simulink model "ensembleSNN_simulink"  (R2019a)
settings: Solver=FixedStepAuto  StartTime=0.0  StopTime=12  FixedStep=0.001  RelTol=1e-3
libraries: simulink x2, dspsigops x1
(part 2 of 3)

== system ensembleSNN_simulink/izhiekvichNeuron10/u' switch ==
  In1 : Inport
  In2 : Inport  Port=2
  In3 : Inport  Port=3
  Switch Delay - 3 : Delay  DelayLength=3
  Switch4 : Switch  Criteria=u2 > Threshold  Threshold=30
  Out1 : Outport  VectorParamsAs1DForOutWhenUnconnected=on
  wires:
  In2/1 -> Switch4/2
  Switch4/1 -> Switch Delay - 3/1
  In1/1 -> Switch4/1
  Switch Delay - 3/1 -> Out1/1
  In3/1 -> Switch4/3

== system ensembleSNN_simulink/izhiekvichNeuron10/v + [0.04v2 +5v - u + j +140 ==
  In1 : Inport
  J : Inport  Port=2
  Add : Sum
  Add Delay - 2 : Delay
  Out1 : Outport  VectorParamsAs1DForOutWhenUnconnected=on
  wires:
  Add Delay - 2/1 -> Out1/1
  Add/1 -> Add Delay - 2/1
  In1/1 -> Add/1
  J/1 -> Add/2

== system ensembleSNN_simulink/izhiekvichNeuron10/v' switch ==
  In1 : Inport
  In2 : Inport  Port=2
  In3 : Inport  Port=3
  Switch Delay - 3 : Delay  DelayLength=3
  Switch4 : Switch  Criteria=u2 > Threshold  Threshold=30
  J : Outport  VectorParamsAs1DForOutWhenUnconnected=on
  wires:
  In2/1 -> Switch4/2
  Switch4/1 -> Switch Delay - 3/1
  In1/1 -> Switch4/1
  Switch Delay - 3/1 -> J/1
  In3/1 -> Switch4/3

== system ensembleSNN_simulink/izhiekvichNeuron10/v^2 ==
  J : Inport
  In2 : Inport  Port=2
  Mult Delay - 2 : Delay  DelayLength=1
  Product1 : Product
  Out1 : Outport  VectorParamsAs1DForOutWhenUnconnected=on
  wires:
  Product1/1 -> Mult Delay - 2/1
  In2/1 -> Product1/2
  J/1 -> Product1/1
  Mult Delay - 2/1 -> Out1/1

== system ensembleSNN_simulink/izhiekvichNeuron11/0.04v2 +5v - u ==
  In1 : Inport
  In2 : Inport  Port=2
  Subtract : Sum  Inputs=+-
  Subtract Delay - 1 : Delay  DelayLength=1
  Out1 : Outport  VectorParamsAs1DForOutWhenUnconnected=on
  wires:
  In1/1 -> Subtract/1
  Subtract/1 -> Subtract Delay - 1/1
  Subtract Delay - 1/1 -> Out1/1
  In2/1 -> Subtract/2

== system ensembleSNN_simulink/izhiekvichNeuron11/0.04v2 +5v - u + j +140 ==
  In1 : Inport
  J : Inport  Port=2
  Add : Sum
  Add Delay - 2 : Delay
  Out1 : Outport  VectorParamsAs1DForOutWhenUnconnected=on
  wires:
  Add Delay - 2/1 -> Out1/1
  Add/1 -> Add Delay - 2/1
  In1/1 -> Add/1
  J/1 -> Add/2

== system ensembleSNN_simulink/izhiekvichNeuron11/0.04v^2 ==
  In1 : Inport
  In2 : Inport  Port=2
  Mult Delay - 1 : Delay  DelayLength=1
  Product1 : Product
  Out1 : Outport  VectorParamsAs1DForOutWhenUnconnected=on
  wires:
  Product1/1 -> Mult Delay - 1/1
  Mult Delay - 1/1 -> Out1/1
  In2/1 -> Product1/2
  In1/1 -> Product1/1

== system ensembleSNN_simulink/izhiekvichNeuron11/0.04v^2 +5v ==
  In1 : Inport
  In2 : Inport  Port=2
  Add : Sum
  Add Delay - 2 : Delay
  Out1 : Outport  VectorParamsAs1DForOutWhenUnconnected=on
  wires:
  Add Delay - 2/1 -> Out1/1
  Add/1 -> Add Delay - 2/1
  In1/1 -> Add/1
  In2/1 -> Add/2

== system ensembleSNN_simulink/izhiekvichNeuron11/5v ==
  J : Inport
  In2 : Inport  Port=2
  Mult Delay - 1 : Delay  DelayLength=1
  Product1 : Product
  Out1 : Outport  VectorParamsAs1DForOutWhenUnconnected=on
  wires:
  Product1/1 -> Mult Delay - 1/1
  Mult Delay - 1/1 -> Out1/1
  In2/1 -> Product1/2
  J/1 -> Product1/1

== system ensembleSNN_simulink/izhiekvichNeuron11/a(bv-u) ==
  In1 : Inport
  In2 : Inport  Port=2
  Mult Delay - 1 : Delay  DelayLength=1
  Product1 : Product
  Out1 : Outport  VectorParamsAs1DForOutWhenUnconnected=on
  wires:
  Product1/1 -> Mult Delay - 1/1
  Mult Delay - 1/1 -> Out1/1
  In2/1 -> Product1/2
  In1/1 -> Product1/1

== system ensembleSNN_simulink/izhiekvichNeuron11/bv ==
  In1 : Inport
  J : Inport  Port=2
  Mult Delay - 1 : Delay  DelayLength=1
  Product1 : Product
  Out1 : Outport  VectorParamsAs1DForOutWhenUnconnected=on
  wires:
  Product1/1 -> Mult Delay - 1/1
  Mult Delay - 1/1 -> Out1/1
  J/1 -> Product1/2
  In1/1 -> Product1/1

== system ensembleSNN_simulink/izhiekvichNeuron11/bv - u ==
  In1 : Inport
  In2 : Inport  Port=2
  Subtract : Sum  Inputs=+-
  Subtract Delay - 1 : Delay  DelayLength=1
  Out1 : Outport  VectorParamsAs1DForOutWhenUnconnected=on
  wires:
  In1/1 -> Subtract/1
  Subtract/1 -> Subtract Delay - 1/1
  Subtract Delay - 1/1 -> Out1/1
  In2/1 -> Subtract/2

== system ensembleSNN_simulink/izhiekvichNeuron11/j + 140 ==
  In1 : Inport
  J : Inport  Port=2
  Add : Sum
  Add Delay - 2 : Delay
  Out1 : Outport  VectorParamsAs1DForOutWhenUnconnected=on
  wires:
  Add Delay - 2/1 -> Out1/1
  Add/1 -> Add Delay - 2/1
  In1/1 -> Add/1
  J/1 -> Add/2

== system ensembleSNN_simulink/izhiekvichNeuron11/u + a(bv-u) ==
  In1 : Inport
  In2 : Inport  Port=2
  Add : Sum
  Add Delay - 2 : Delay
  Out1 : Outport  VectorParamsAs1DForOutWhenUnconnected=on
  wires:
  Add Delay - 2/1 -> Out1/1
  Add/1 -> Add Delay - 2/1
  In1/1 -> Add/1
  In2/1 -> Add/2

== system ensembleSNN_simulink/izhiekvichNeuron11/u' + d ==
  In1 : Inport
  In2 : Inport  Port=2
  Add : Sum
  Add Delay - 2 : Delay
  Out1 : Outport  VectorParamsAs1DForOutWhenUnconnected=on
  wires:
  Add Delay - 2/1 -> Out1/1
  Add/1 -> Add Delay - 2/1
  In1/1 -> Add/1
  In2/1 -> Add/2

== system ensembleSNN_simulink/izhiekvichNeuron11/u' switch ==
  In1 : Inport
  In2 : Inport  Port=2
  In3 : Inport  Port=3
  Switch Delay - 3 : Delay  DelayLength=3
  Switch4 : Switch  Criteria=u2 > Threshold  Threshold=30
  Out1 : Outport  VectorParamsAs1DForOutWhenUnconnected=on
  wires:
  In2/1 -> Switch4/2
  Switch4/1 -> Switch Delay - 3/1
  In1/1 -> Switch4/1
  Switch Delay - 3/1 -> Out1/1
  In3/1 -> Switch4/3

== system ensembleSNN_simulink/izhiekvichNeuron11/v + [0.04v2 +5v - u + j +140 ==
  In1 : Inport
  J : Inport  Port=2
  Add : Sum
  Add Delay - 2 : Delay
  Out1 : Outport  VectorParamsAs1DForOutWhenUnconnected=on
  wires:
  Add Delay - 2/1 -> Out1/1
  Add/1 -> Add Delay - 2/1
  In1/1 -> Add/1
  J/1 -> Add/2

== system ensembleSNN_simulink/izhiekvichNeuron11/v' switch ==
  In1 : Inport
  In2 : Inport  Port=2
  In3 : Inport  Port=3
  Switch Delay - 3 : Delay  DelayLength=3
  Switch4 : Switch  Criteria=u2 > Threshold  Threshold=30
  J : Outport  VectorParamsAs1DForOutWhenUnconnected=on
  wires:
  In2/1 -> Switch4/2
  Switch4/1 -> Switch Delay - 3/1
  In1/1 -> Switch4/1
  Switch Delay - 3/1 -> J/1
  In3/1 -> Switch4/3

== system ensembleSNN_simulink/izhiekvichNeuron11/v^2 ==
  J : Inport
  In2 : Inport  Port=2
  Mult Delay - 2 : Delay  DelayLength=1
  Product1 : Product
  Out1 : Outport  VectorParamsAs1DForOutWhenUnconnected=on
  wires:
  Product1/1 -> Mult Delay - 2/1
  In2/1 -> Product1/2
  J/1 -> Product1/1
  Mult Delay - 2/1 -> Out1/1

== system ensembleSNN_simulink/izhiekvichNeuron12/0.04v2 +5v - u ==
  In1 : Inport
  In2 : Inport  Port=2
  Subtract : Sum  Inputs=+-
  Subtract Delay - 1 : Delay  DelayLength=1
  Out1 : Outport  VectorParamsAs1DForOutWhenUnconnected=on
  wires:
  In1/1 -> Subtract/1
  Subtract/1 -> Subtract Delay - 1/1
  Subtract Delay - 1/1 -> Out1/1
  In2/1 -> Subtract/2

== system ensembleSNN_simulink/izhiekvichNeuron12/0.04v2 +5v - u + j +140 ==
  In1 : Inport
  J : Inport  Port=2
  Add : Sum
  Add Delay - 2 : Delay
  Out1 : Outport  VectorParamsAs1DForOutWhenUnconnected=on
  wires:
  Add Delay - 2/1 -> Out1/1
  Add/1 -> Add Delay - 2/1
  In1/1 -> Add/1
  J/1 -> Add/2

== system ensembleSNN_simulink/izhiekvichNeuron12/0.04v^2 ==
  In1 : Inport
  In2 : Inport  Port=2
  Mult Delay - 1 : Delay  DelayLength=1
  Product1 : Product
  Out1 : Outport  VectorParamsAs1DForOutWhenUnconnected=on
  wires:
  Product1/1 -> Mult Delay - 1/1
  Mult Delay - 1/1 -> Out1/1
  In2/1 -> Product1/2
  In1/1 -> Product1/1

== system ensembleSNN_simulink/izhiekvichNeuron12/0.04v^2 +5v ==
  In1 : Inport
  In2 : Inport  Port=2
  Add : Sum
  Add Delay - 2 : Delay
  Out1 : Outport  VectorParamsAs1DForOutWhenUnconnected=on
  wires:
  Add Delay - 2/1 -> Out1/1
  Add/1 -> Add Delay - 2/1
  In1/1 -> Add/1
  In2/1 -> Add/2

== system ensembleSNN_simulink/izhiekvichNeuron12/5v ==
  J : Inport
  In2 : Inport  Port=2
  Mult Delay - 1 : Delay  DelayLength=1
  Product1 : Product
  Out1 : Outport  VectorParamsAs1DForOutWhenUnconnected=on
  wires:
  Product1/1 -> Mult Delay - 1/1
  Mult Delay - 1/1 -> Out1/1
  In2/1 -> Product1/2
  J/1 -> Product1/1

== system ensembleSNN_simulink/izhiekvichNeuron12/a(bv-u) ==
  In1 : Inport
  In2 : Inport  Port=2
  Mult Delay - 1 : Delay  DelayLength=1
  Product1 : Product
  Out1 : Outport  VectorParamsAs1DForOutWhenUnconnected=on
  wires:
  Product1/1 -> Mult Delay - 1/1
  Mult Delay - 1/1 -> Out1/1
  In2/1 -> Product1/2
  In1/1 -> Product1/1

== system ensembleSNN_simulink/izhiekvichNeuron12/bv ==
  In1 : Inport
  J : Inport  Port=2
  Mult Delay - 1 : Delay  DelayLength=1
  Product1 : Product
  Out1 : Outport  VectorParamsAs1DForOutWhenUnconnected=on
  wires:
  Product1/1 -> Mult Delay - 1/1
  Mult Delay - 1/1 -> Out1/1
  J/1 -> Product1/2
  In1/1 -> Product1/1

== system ensembleSNN_simulink/izhiekvichNeuron12/bv - u ==
  In1 : Inport
  In2 : Inport  Port=2
  Subtract : Sum  Inputs=+-
  Subtract Delay - 1 : Delay  DelayLength=1
  Out1 : Outport  VectorParamsAs1DForOutWhenUnconnected=on
  wires:
  In1/1 -> Subtract/1
  Subtract/1 -> Subtract Delay - 1/1
  Subtract Delay - 1/1 -> Out1/1
  In2/1 -> Subtract/2

== system ensembleSNN_simulink/izhiekvichNeuron12/j + 140 ==
  In1 : Inport
  J : Inport  Port=2
  Add : Sum
  Add Delay - 2 : Delay
  Out1 : Outport  VectorParamsAs1DForOutWhenUnconnected=on
  wires:
  Add Delay - 2/1 -> Out1/1
  Add/1 -> Add Delay - 2/1
  In1/1 -> Add/1
  J/1 -> Add/2

== system ensembleSNN_simulink/izhiekvichNeuron12/u + a(bv-u) ==
  In1 : Inport
  In2 : Inport  Port=2
  Add : Sum
  Add Delay - 2 : Delay
  Out1 : Outport  VectorParamsAs1DForOutWhenUnconnected=on
  wires:
  Add Delay - 2/1 -> Out1/1
  Add/1 -> Add Delay - 2/1
  In1/1 -> Add/1
  In2/1 -> Add/2

== system ensembleSNN_simulink/izhiekvichNeuron12/u' + d ==
  In1 : Inport
  In2 : Inport  Port=2
  Add : Sum
  Add Delay - 2 : Delay
  Out1 : Outport  VectorParamsAs1DForOutWhenUnconnected=on
  wires:
  Add Delay - 2/1 -> Out1/1
  Add/1 -> Add Delay - 2/1
  In1/1 -> Add/1
  In2/1 -> Add/2

== system ensembleSNN_simulink/izhiekvichNeuron12/u' switch ==
  In1 : Inport
  In2 : Inport  Port=2
  In3 : Inport  Port=3
  Switch Delay - 3 : Delay  DelayLength=3
  Switch4 : Switch  Criteria=u2 > Threshold  Threshold=30
  Out1 : Outport  VectorParamsAs1DForOutWhenUnconnected=on
  wires:
  In2/1 -> Switch4/2
  Switch4/1 -> Switch Delay - 3/1
  In1/1 -> Switch4/1
  Switch Delay - 3/1 -> Out1/1
  In3/1 -> Switch4/3

== system ensembleSNN_simulink/izhiekvichNeuron12/v + [0.04v2 +5v - u + j +140 ==
  In1 : Inport
  J : Inport  Port=2
  Add : Sum
  Add Delay - 2 : Delay
  Out1 : Outport  VectorParamsAs1DForOutWhenUnconnected=on
  wires:
  Add Delay - 2/1 -> Out1/1
  Add/1 -> Add Delay - 2/1
  In1/1 -> Add/1
  J/1 -> Add/2

== system ensembleSNN_simulink/izhiekvichNeuron12/v' switch ==
  In1 : Inport
  In2 : Inport  Port=2
  In3 : Inport  Port=3
  Switch Delay - 3 : Delay  DelayLength=3
  Switch4 : Switch  Criteria=u2 > Threshold  Threshold=30
  J : Outport  VectorParamsAs1DForOutWhenUnconnected=on
  wires:
  In2/1 -> Switch4/2
  Switch4/1 -> Switch Delay - 3/1
  In1/1 -> Switch4/1
  Switch Delay - 3/1 -> J/1
  In3/1 -> Switch4/3

== system ensembleSNN_simulink/izhiekvichNeuron12/v^2 ==
  J : Inport
  In2 : Inport  Port=2
  Mult Delay - 2 : Delay  DelayLength=1
  Product1 : Product
  Out1 : Outport  VectorParamsAs1DForOutWhenUnconnected=on
  wires:
  Product1/1 -> Mult Delay - 2/1
  In2/1 -> Product1/2
  J/1 -> Product1/1
  Mult Delay - 2/1 -> Out1/1

== system ensembleSNN_simulink/izhiekvichNeuron13/0.04v2 +5v - u ==
  In1 : Inport
  In2 : Inport  Port=2
  Subtract : Sum  Inputs=+-
  Subtract Delay - 1 : Delay  DelayLength=1
  Out1 : Outport  VectorParamsAs1DForOutWhenUnconnected=on
  wires:
  In1/1 -> Subtract/1
  Subtract/1 -> Subtract Delay - 1/1
  Subtract Delay - 1/1 -> Out1/1
  In2/1 -> Subtract/2

== system ensembleSNN_simulink/izhiekvichNeuron13/0.04v2 +5v - u + j +140 ==
  In1 : Inport
  J : Inport  Port=2
  Add : Sum
  Add Delay - 2 : Delay
  Out1 : Outport  VectorParamsAs1DForOutWhenUnconnected=on
  wires:
  Add Delay - 2/1 -> Out1/1
  Add/1 -> Add Delay - 2/1
  In1/1 -> Add/1
  J/1 -> Add/2

== system ensembleSNN_simulink/izhiekvichNeuron13/0.04v^2 ==
  In1 : Inport
  In2 : Inport  Port=2
  Mult Delay - 1 : Delay  DelayLength=1
  Product1 : Product
  Out1 : Outport  VectorParamsAs1DForOutWhenUnconnected=on
  wires:
  Product1/1 -> Mult Delay - 1/1
  Mult Delay - 1/1 -> Out1/1
  In2/1 -> Product1/2
  In1/1 -> Product1/1

== system ensembleSNN_simulink/izhiekvichNeuron13/0.04v^2 +5v ==
  In1 : Inport
  In2 : Inport  Port=2
  Add : Sum
  Add Delay - 2 : Delay
  Out1 : Outport  VectorParamsAs1DForOutWhenUnconnected=on
  wires:
  Add Delay - 2/1 -> Out1/1
  Add/1 -> Add Delay - 2/1
  In1/1 -> Add/1
  In2/1 -> Add/2

== system ensembleSNN_simulink/izhiekvichNeuron13/5v ==
  J : Inport
  In2 : Inport  Port=2
  Mult Delay - 1 : Delay  DelayLength=1
  Product1 : Product
  Out1 : Outport  VectorParamsAs1DForOutWhenUnconnected=on
  wires:
  Product1/1 -> Mult Delay - 1/1
  Mult Delay - 1/1 -> Out1/1
  In2/1 -> Product1/2
  J/1 -> Product1/1

== system ensembleSNN_simulink/izhiekvichNeuron13/a(bv-u) ==
  In1 : Inport
  In2 : Inport  Port=2
  Mult Delay - 1 : Delay  DelayLength=1
  Product1 : Product
  Out1 : Outport  VectorParamsAs1DForOutWhenUnconnected=on
  wires:
  Product1/1 -> Mult Delay - 1/1
  Mult Delay - 1/1 -> Out1/1
  In2/1 -> Product1/2
  In1/1 -> Product1/1

== system ensembleSNN_simulink/izhiekvichNeuron13/bv ==
  In1 : Inport
  J : Inport  Port=2
  Mult Delay - 1 : Delay  DelayLength=1
  Product1 : Product
  Out1 : Outport  VectorParamsAs1DForOutWhenUnconnected=on
  wires:
  Product1/1 -> Mult Delay - 1/1
  Mult Delay - 1/1 -> Out1/1
  J/1 -> Product1/2
  In1/1 -> Product1/1

== system ensembleSNN_simulink/izhiekvichNeuron13/bv - u ==
  In1 : Inport
  In2 : Inport  Port=2
  Subtract : Sum  Inputs=+-
  Subtract Delay - 1 : Delay  DelayLength=1
  Out1 : Outport  VectorParamsAs1DForOutWhenUnconnected=on
  wires:
  In1/1 -> Subtract/1
  Subtract/1 -> Subtract Delay - 1/1
  Subtract Delay - 1/1 -> Out1/1
  In2/1 -> Subtract/2

== system ensembleSNN_simulink/izhiekvichNeuron13/j + 140 ==
  In1 : Inport
  J : Inport  Port=2
  Add : Sum
  Add Delay - 2 : Delay
  Out1 : Outport  VectorParamsAs1DForOutWhenUnconnected=on
  wires:
  Add Delay - 2/1 -> Out1/1
  Add/1 -> Add Delay - 2/1
  In1/1 -> Add/1
  J/1 -> Add/2

== system ensembleSNN_simulink/izhiekvichNeuron13/u + a(bv-u) ==
  In1 : Inport
  In2 : Inport  Port=2
  Add : Sum
  Add Delay - 2 : Delay
  Out1 : Outport  VectorParamsAs1DForOutWhenUnconnected=on
  wires:
  Add Delay - 2/1 -> Out1/1
  Add/1 -> Add Delay - 2/1
  In1/1 -> Add/1
  In2/1 -> Add/2

== system ensembleSNN_simulink/izhiekvichNeuron13/u' + d ==
  In1 : Inport
  In2 : Inport  Port=2
  Add : Sum
  Add Delay - 2 : Delay
  Out1 : Outport  VectorParamsAs1DForOutWhenUnconnected=on
  wires:
  Add Delay - 2/1 -> Out1/1
  Add/1 -> Add Delay - 2/1
  In1/1 -> Add/1
  In2/1 -> Add/2

== system ensembleSNN_simulink/izhiekvichNeuron13/u' switch ==
  In1 : Inport
  In2 : Inport  Port=2
  In3 : Inport  Port=3
  Switch Delay - 3 : Delay  DelayLength=3
  Switch4 : Switch  Criteria=u2 > Threshold  Threshold=30
  Out1 : Outport  VectorParamsAs1DForOutWhenUnconnected=on
  wires:
  In2/1 -> Switch4/2
  Switch4/1 -> Switch Delay - 3/1
  In1/1 -> Switch4/1
  Switch Delay - 3/1 -> Out1/1
  In3/1 -> Switch4/3

== system ensembleSNN_simulink/izhiekvichNeuron13/v + [0.04v2 +5v - u + j +140 ==
  In1 : Inport
  J : Inport  Port=2
  Add : Sum
  Add Delay - 2 : Delay
  Out1 : Outport  VectorParamsAs1DForOutWhenUnconnected=on
  wires:
  Add Delay - 2/1 -> Out1/1
  Add/1 -> Add Delay - 2/1
  In1/1 -> Add/1
  J/1 -> Add/2

== system ensembleSNN_simulink/izhiekvichNeuron13/v' switch ==
  In1 : Inport
  In2 : Inport  Port=2
  In3 : Inport  Port=3
  Switch Delay - 3 : Delay  DelayLength=3
  Switch4 : Switch  Criteria=u2 > Threshold  Threshold=30
  J : Outport  VectorParamsAs1DForOutWhenUnconnected=on
  wires:
  In2/1 -> Switch4/2
  Switch4/1 -> Switch Delay - 3/1
  In1/1 -> Switch4/1
  Switch Delay - 3/1 -> J/1
  In3/1 -> Switch4/3

== system ensembleSNN_simulink/izhiekvichNeuron13/v^2 ==
  J : Inport
  In2 : Inport  Port=2
  Mult Delay - 2 : Delay  DelayLength=1
  Product1 : Product
  Out1 : Outport  VectorParamsAs1DForOutWhenUnconnected=on
  wires:
  Product1/1 -> Mult Delay - 2/1
  In2/1 -> Product1/2
  J/1 -> Product1/1
  Mult Delay - 2/1 -> Out1/1

== system ensembleSNN_simulink/izhiekvichNeuron14/0.04v2 +5v - u ==
  In1 : Inport
  In2 : Inport  Port=2
  Subtract : Sum  Inputs=+-
  Subtract Delay - 1 : Delay  DelayLength=1
  Out1 : Outport  VectorParamsAs1DForOutWhenUnconnected=on
  wires:
  In1/1 -> Subtract/1
  Subtract/1 -> Subtract Delay - 1/1
  Subtract Delay - 1/1 -> Out1/1
  In2/1 -> Subtract/2

== system ensembleSNN_simulink/izhiekvichNeuron14/0.04v2 +5v - u + j +140 ==
  In1 : Inport
  J : Inport  Port=2
  Add : Sum
  Add Delay - 2 : Delay
  Out1 : Outport  VectorParamsAs1DForOutWhenUnconnected=on
  wires:
  Add Delay - 2/1 -> Out1/1
  Add/1 -> Add Delay - 2/1
  In1/1 -> Add/1
  J/1 -> Add/2

== system ensembleSNN_simulink/izhiekvichNeuron14/0.04v^2 ==
  In1 : Inport
  In2 : Inport  Port=2
  Mult Delay - 1 : Delay  DelayLength=1
  Product1 : Product
  Out1 : Outport  VectorParamsAs1DForOutWhenUnconnected=on
  wires:
  Product1/1 -> Mult Delay - 1/1
  Mult Delay - 1/1 -> Out1/1
  In2/1 -> Product1/2
  In1/1 -> Product1/1

== system ensembleSNN_simulink/izhiekvichNeuron14/0.04v^2 +5v ==
  In1 : Inport
  In2 : Inport  Port=2
  Add : Sum
  Add Delay - 2 : Delay
  Out1 : Outport  VectorParamsAs1DForOutWhenUnconnected=on
  wires:
  Add Delay - 2/1 -> Out1/1
  Add/1 -> Add Delay - 2/1
  In1/1 -> Add/1
  In2/1 -> Add/2

== system ensembleSNN_simulink/izhiekvichNeuron14/5v ==
  J : Inport
  In2 : Inport  Port=2
  Mult Delay - 1 : Delay  DelayLength=1
  Product1 : Product
  Out1 : Outport  VectorParamsAs1DForOutWhenUnconnected=on
  wires:
  Product1/1 -> Mult Delay - 1/1
  Mult Delay - 1/1 -> Out1/1
  In2/1 -> Product1/2
  J/1 -> Product1/1

== system ensembleSNN_simulink/izhiekvichNeuron14/a(bv-u) ==
  In1 : Inport
  In2 : Inport  Port=2
  Mult Delay - 1 : Delay  DelayLength=1
  Product1 : Product
  Out1 : Outport  VectorParamsAs1DForOutWhenUnconnected=on
  wires:
  Product1/1 -> Mult Delay - 1/1
  Mult Delay - 1/1 -> Out1/1
  In2/1 -> Product1/2
  In1/1 -> Product1/1

== system ensembleSNN_simulink/izhiekvichNeuron14/bv ==
  In1 : Inport
  J : Inport  Port=2
  Mult Delay - 1 : Delay  DelayLength=1
  Product1 : Product
  Out1 : Outport  VectorParamsAs1DForOutWhenUnconnected=on
  wires:
  Product1/1 -> Mult Delay - 1/1
  Mult Delay - 1/1 -> Out1/1
  J/1 -> Product1/2
  In1/1 -> Product1/1

== system ensembleSNN_simulink/izhiekvichNeuron14/bv - u ==
  In1 : Inport
  In2 : Inport  Port=2
  Subtract : Sum  Inputs=+-
  Subtract Delay - 1 : Delay  DelayLength=1
  Out1 : Outport  VectorParamsAs1DForOutWhenUnconnected=on
  wires:
  In1/1 -> Subtract/1
  Subtract/1 -> Subtract Delay - 1/1
  Subtract Delay - 1/1 -> Out1/1
  In2/1 -> Subtract/2

== system ensembleSNN_simulink/izhiekvichNeuron14/j + 140 ==
  In1 : Inport
  J : Inport  Port=2
  Add : Sum
  Add Delay - 2 : Delay
  Out1 : Outport  VectorParamsAs1DForOutWhenUnconnected=on
  wires:
  Add Delay - 2/1 -> Out1/1
  Add/1 -> Add Delay - 2/1
  In1/1 -> Add/1
  J/1 -> Add/2

== system ensembleSNN_simulink/izhiekvichNeuron14/u + a(bv-u) ==
  In1 : Inport
  In2 : Inport  Port=2
  Add : Sum
  Add Delay - 2 : Delay
  Out1 : Outport  VectorParamsAs1DForOutWhenUnconnected=on
  wires:
  Add Delay - 2/1 -> Out1/1
  Add/1 -> Add Delay - 2/1
  In1/1 -> Add/1
  In2/1 -> Add/2

== system ensembleSNN_simulink/izhiekvichNeuron14/u' + d ==
  In1 : Inport
  In2 : Inport  Port=2
  Add : Sum
  Add Delay - 2 : Delay
  Out1 : Outport  VectorParamsAs1DForOutWhenUnconnected=on
  wires:
  Add Delay - 2/1 -> Out1/1
  Add/1 -> Add Delay - 2/1
  In1/1 -> Add/1
  In2/1 -> Add/2

== system ensembleSNN_simulink/izhiekvichNeuron14/u' switch ==
  In1 : Inport
  In2 : Inport  Port=2
  In3 : Inport  Port=3
  Switch Delay - 3 : Delay  DelayLength=3
  Switch4 : Switch  Criteria=u2 > Threshold  Threshold=30
  Out1 : Outport  VectorParamsAs1DForOutWhenUnconnected=on
  wires:
  In2/1 -> Switch4/2
  Switch4/1 -> Switch Delay - 3/1
  In1/1 -> Switch4/1
  Switch Delay - 3/1 -> Out1/1
  In3/1 -> Switch4/3

== system ensembleSNN_simulink/izhiekvichNeuron14/v + [0.04v2 +5v - u + j +140 ==
  In1 : Inport
  J : Inport  Port=2
  Add : Sum
  Add Delay - 2 : Delay
  Out1 : Outport  VectorParamsAs1DForOutWhenUnconnected=on
  wires:
  Add Delay - 2/1 -> Out1/1
  Add/1 -> Add Delay - 2/1
  In1/1 -> Add/1
  J/1 -> Add/2

== system ensembleSNN_simulink/izhiekvichNeuron14/v' switch ==
  In1 : Inport
  In2 : Inport  Port=2
  In3 : Inport  Port=3
  Switch Delay - 3 : Delay  DelayLength=3
  Switch4 : Switch  Criteria=u2 > Threshold  Threshold=30
  J : Outport  VectorParamsAs1DForOutWhenUnconnected=on
  wires:
  In2/1 -> Switch4/2
  Switch4/1 -> Switch Delay - 3/1
  In1/1 -> Switch4/1
  Switch Delay - 3/1 -> J/1
  In3/1 -> Switch4/3

== system ensembleSNN_simulink/izhiekvichNeuron14/v^2 ==
  J : Inport
  In2 : Inport  Port=2
  Mult Delay - 2 : Delay  DelayLength=1
  Product1 : Product
  Out1 : Outport  VectorParamsAs1DForOutWhenUnconnected=on
  wires:
  Product1/1 -> Mult Delay - 2/1
  In2/1 -> Product1/2
  J/1 -> Product1/1
  Mult Delay - 2/1 -> Out1/1

== system ensembleSNN_simulink/izhiekvichNeuron15/0.04v2 +5v - u ==
  In1 : Inport
  In2 : Inport  Port=2
  Subtract : Sum  Inputs=+-
  Subtract Delay - 1 : Delay  DelayLength=1
  Out1 : Outport  VectorParamsAs1DForOutWhenUnconnected=on
  wires:
  In1/1 -> Subtract/1
  Subtract/1 -> Subtract Delay - 1/1
  Subtract Delay - 1/1 -> Out1/1
  In2/1 -> Subtract/2

== system ensembleSNN_simulink/izhiekvichNeuron15/0.04v2 +5v - u + j +140 ==
  In1 : Inport
  J : Inport  Port=2
  Add : Sum
  Add Delay - 2 : Delay
  Out1 : Outport  VectorParamsAs1DForOutWhenUnconnected=on
  wires:
  Add Delay - 2/1 -> Out1/1
  Add/1 -> Add Delay - 2/1
  In1/1 -> Add/1
  J/1 -> Add/2

== system ensembleSNN_simulink/izhiekvichNeuron15/0.04v^2 ==
  In1 : Inport
  In2 : Inport  Port=2
  Mult Delay - 1 : Delay  DelayLength=1
  Product1 : Product
  Out1 : Outport  VectorParamsAs1DForOutWhenUnconnected=on
  wires:
  Product1/1 -> Mult Delay - 1/1
  Mult Delay - 1/1 -> Out1/1
  In2/1 -> Product1/2
  In1/1 -> Product1/1

== system ensembleSNN_simulink/izhiekvichNeuron15/0.04v^2 +5v ==
  In1 : Inport
  In2 : Inport  Port=2
  Add : Sum
  Add Delay - 2 : Delay
  Out1 : Outport  VectorParamsAs1DForOutWhenUnconnected=on
  wires:
  Add Delay - 2/1 -> Out1/1
  Add/1 -> Add Delay - 2/1
  In1/1 -> Add/1
  In2/1 -> Add/2

== system ensembleSNN_simulink/izhiekvichNeuron15/5v ==
  J : Inport
  In2 : Inport  Port=2
  Mult Delay - 1 : Delay  DelayLength=1
  Product1 : Product
  Out1 : Outport  VectorParamsAs1DForOutWhenUnconnected=on
  wires:
  Product1/1 -> Mult Delay - 1/1
  Mult Delay - 1/1 -> Out1/1
  In2/1 -> Product1/2
  J/1 -> Product1/1

== system ensembleSNN_simulink/izhiekvichNeuron15/a(bv-u) ==
  In1 : Inport
  In2 : Inport  Port=2
  Mult Delay - 1 : Delay  DelayLength=1
  Product1 : Product
  Out1 : Outport  VectorParamsAs1DForOutWhenUnconnected=on
  wires:
  Product1/1 -> Mult Delay - 1/1
  Mult Delay - 1/1 -> Out1/1
  In2/1 -> Product1/2
  In1/1 -> Product1/1

== system ensembleSNN_simulink/izhiekvichNeuron15/bv ==
  In1 : Inport
  J : Inport  Port=2
  Mult Delay - 1 : Delay  DelayLength=1
  Product1 : Product
  Out1 : Outport  VectorParamsAs1DForOutWhenUnconnected=on
  wires:
  Product1/1 -> Mult Delay - 1/1
  Mult Delay - 1/1 -> Out1/1
  J/1 -> Product1/2
  In1/1 -> Product1/1

== system ensembleSNN_simulink/izhiekvichNeuron15/bv - u ==
  In1 : Inport
  In2 : Inport  Port=2
  Subtract : Sum  Inputs=+-
  Subtract Delay - 1 : Delay  DelayLength=1
  Out1 : Outport  VectorParamsAs1DForOutWhenUnconnected=on
  wires:
  In1/1 -> Subtract/1
  Subtract/1 -> Subtract Delay - 1/1
  Subtract Delay - 1/1 -> Out1/1
  In2/1 -> Subtract/2

== system ensembleSNN_simulink/izhiekvichNeuron15/j + 140 ==
  In1 : Inport
  J : Inport  Port=2
  Add : Sum
  Add Delay - 2 : Delay
  Out1 : Outport  VectorParamsAs1DForOutWhenUnconnected=on
  wires:
  Add Delay - 2/1 -> Out1/1
  Add/1 -> Add Delay - 2/1
  In1/1 -> Add/1
  J/1 -> Add/2

== system ensembleSNN_simulink/izhiekvichNeuron15/u + a(bv-u) ==
  In1 : Inport
  In2 : Inport  Port=2
  Add : Sum
  Add Delay - 2 : Delay
  Out1 : Outport  VectorParamsAs1DForOutWhenUnconnected=on
  wires:
  Add Delay - 2/1 -> Out1/1
  Add/1 -> Add Delay - 2/1
  In1/1 -> Add/1
  In2/1 -> Add/2

== system ensembleSNN_simulink/izhiekvichNeuron15/u' + d ==
  In1 : Inport
  In2 : Inport  Port=2
  Add : Sum
  Add Delay - 2 : Delay
  Out1 : Outport  VectorParamsAs1DForOutWhenUnconnected=on
  wires:
  Add Delay - 2/1 -> Out1/1
  Add/1 -> Add Delay - 2/1
  In1/1 -> Add/1
  In2/1 -> Add/2

== system ensembleSNN_simulink/izhiekvichNeuron15/u' switch ==
  In1 : Inport
  In2 : Inport  Port=2
  In3 : Inport  Port=3
  Switch Delay - 3 : Delay  DelayLength=3
  Switch4 : Switch  Criteria=u2 > Threshold  Threshold=30
  Out1 : Outport  VectorParamsAs1DForOutWhenUnconnected=on
  wires:
  In2/1 -> Switch4/2
  Switch4/1 -> Switch Delay - 3/1
  In1/1 -> Switch4/1
  Switch Delay - 3/1 -> Out1/1
  In3/1 -> Switch4/3

== system ensembleSNN_simulink/izhiekvichNeuron15/v + [0.04v2 +5v - u + j +140 ==
  In1 : Inport
  J : Inport  Port=2
  Add : Sum
  Add Delay - 2 : Delay
  Out1 : Outport  VectorParamsAs1DForOutWhenUnconnected=on
  wires:
  Add Delay - 2/1 -> Out1/1
  Add/1 -> Add Delay - 2/1
  In1/1 -> Add/1
  J/1 -> Add/2

== system ensembleSNN_simulink/izhiekvichNeuron15/v' switch ==
  In1 : Inport
  In2 : Inport  Port=2
  In3 : Inport  Port=3
  Switch Delay - 3 : Delay  DelayLength=3
  Switch4 : Switch  Criteria=u2 > Threshold  Threshold=30
  J : Outport  VectorParamsAs1DForOutWhenUnconnected=on
  wires:
  In2/1 -> Switch4/2
  Switch4/1 -> Switch Delay - 3/1
  In1/1 -> Switch4/1
  Switch Delay - 3/1 -> J/1
  In3/1 -> Switch4/3

== system ensembleSNN_simulink/izhiekvichNeuron15/v^2 ==
  J : Inport
  In2 : Inport  Port=2
  Mult Delay - 2 : Delay  DelayLength=1
  Product1 : Product
  Out1 : Outport  VectorParamsAs1DForOutWhenUnconnected=on
  wires:
  Product1/1 -> Mult Delay - 2/1
  In2/1 -> Product1/2
  J/1 -> Product1/1
  Mult Delay - 2/1 -> Out1/1

== system ensembleSNN_simulink/izhiekvichNeuron2/0.04v2 +5v - u ==
  In1 : Inport
  In2 : Inport  Port=2
  Subtract : Sum  Inputs=+-
  Subtract Delay - 1 : Delay  DelayLength=1
  Out1 : Outport  VectorParamsAs1DForOutWhenUnconnected=on
  wires:
  In1/1 -> Subtract/1
  Subtract/1 -> Subtract Delay - 1/1
  Subtract Delay - 1/1 -> Out1/1
  In2/1 -> Subtract/2

== system ensembleSNN_simulink/izhiekvichNeuron2/0.04v2 +5v - u + j +140 ==
  In1 : Inport
  J : Inport  Port=2
  Add : Sum
  Add Delay - 2 : Delay
  Out1 : Outport  VectorParamsAs1DForOutWhenUnconnected=on
  wires:
  Add Delay - 2/1 -> Out1/1
  Add/1 -> Add Delay - 2/1
  In1/1 -> Add/1
  J/1 -> Add/2

== system ensembleSNN_simulink/izhiekvichNeuron2/0.04v^2 ==
  In1 : Inport
  In2 : Inport  Port=2
  Mult Delay - 1 : Delay  DelayLength=1
  Product1 : Product
  Out1 : Outport  VectorParamsAs1DForOutWhenUnconnected=on
  wires:
  Product1/1 -> Mult Delay - 1/1
  Mult Delay - 1/1 -> Out1/1
  In2/1 -> Product1/2
  In1/1 -> Product1/1

== system ensembleSNN_simulink/izhiekvichNeuron2/0.04v^2 +5v ==
  In1 : Inport
  In2 : Inport  Port=2
  Add : Sum
  Add Delay - 2 : Delay
  Out1 : Outport  VectorParamsAs1DForOutWhenUnconnected=on
  wires:
  Add Delay - 2/1 -> Out1/1
  Add/1 -> Add Delay - 2/1
  In1/1 -> Add/1
  In2/1 -> Add/2

== system ensembleSNN_simulink/izhiekvichNeuron2/5v ==
  J : Inport
  In2 : Inport  Port=2
  Mult Delay - 1 : Delay  DelayLength=1
  Product1 : Product
  Out1 : Outport  VectorParamsAs1DForOutWhenUnconnected=on
  wires:
  Product1/1 -> Mult Delay - 1/1
  Mult Delay - 1/1 -> Out1/1
  In2/1 -> Product1/2
  J/1 -> Product1/1

== system ensembleSNN_simulink/izhiekvichNeuron2/a(bv-u) ==
  In1 : Inport
  In2 : Inport  Port=2
  Mult Delay - 1 : Delay  DelayLength=1
  Product1 : Product
  Out1 : Outport  VectorParamsAs1DForOutWhenUnconnected=on
  wires:
  Product1/1 -> Mult Delay - 1/1
  Mult Delay - 1/1 -> Out1/1
  In2/1 -> Product1/2
  In1/1 -> Product1/1

== system ensembleSNN_simulink/izhiekvichNeuron2/bv ==
  In1 : Inport
  J : Inport  Port=2
  Mult Delay - 1 : Delay  DelayLength=1
  Product1 : Product
  Out1 : Outport  VectorParamsAs1DForOutWhenUnconnected=on
  wires:
  Product1/1 -> Mult Delay - 1/1
  Mult Delay - 1/1 -> Out1/1
  J/1 -> Product1/2
  In1/1 -> Product1/1

== system ensembleSNN_simulink/izhiekvichNeuron2/bv - u ==
  In1 : Inport
  In2 : Inport  Port=2
  Subtract : Sum  Inputs=+-
  Subtract Delay - 1 : Delay  DelayLength=1
  Out1 : Outport  VectorParamsAs1DForOutWhenUnconnected=on
  wires:
  In1/1 -> Subtract/1
  Subtract/1 -> Subtract Delay - 1/1
  Subtract Delay - 1/1 -> Out1/1
  In2/1 -> Subtract/2

== system ensembleSNN_simulink/izhiekvichNeuron2/j + 140 ==
  In1 : Inport
  J : Inport  Port=2
  Add : Sum
  Add Delay - 2 : Delay
  Out1 : Outport  VectorParamsAs1DForOutWhenUnconnected=on
  wires:
  Add Delay - 2/1 -> Out1/1
  Add/1 -> Add Delay - 2/1
  In1/1 -> Add/1
  J/1 -> Add/2

== system ensembleSNN_simulink/izhiekvichNeuron2/u + a(bv-u) ==
  In1 : Inport
  In2 : Inport  Port=2
  Add : Sum
  Add Delay - 2 : Delay
  Out1 : Outport  VectorParamsAs1DForOutWhenUnconnected=on
  wires:
  Add Delay - 2/1 -> Out1/1
  Add/1 -> Add Delay - 2/1
  In1/1 -> Add/1
  In2/1 -> Add/2

== system ensembleSNN_simulink/izhiekvichNeuron2/u' + d ==
  In1 : Inport
  In2 : Inport  Port=2
  Add : Sum
  Add Delay - 2 : Delay
  Out1 : Outport  VectorParamsAs1DForOutWhenUnconnected=on
  wires:
  Add Delay - 2/1 -> Out1/1
  Add/1 -> Add Delay - 2/1
  In1/1 -> Add/1
  In2/1 -> Add/2

== system ensembleSNN_simulink/izhiekvichNeuron2/u' switch ==
  In1 : Inport
  In2 : Inport  Port=2
  In3 : Inport  Port=3
  Switch Delay - 3 : Delay  DelayLength=3
  Switch4 : Switch  Criteria=u2 > Threshold  Threshold=30
  Out1 : Outport  VectorParamsAs1DForOutWhenUnconnected=on
  wires:
  In2/1 -> Switch4/2
  Switch4/1 -> Switch Delay - 3/1
  In1/1 -> Switch4/1
  Switch Delay - 3/1 -> Out1/1
  In3/1 -> Switch4/3

== system ensembleSNN_simulink/izhiekvichNeuron2/v + [0.04v2 +5v - u + j +140 ==
  In1 : Inport
  J : Inport  Port=2
  Add : Sum
  Add Delay - 2 : Delay
  Out1 : Outport  VectorParamsAs1DForOutWhenUnconnected=on
  wires:
  Add Delay - 2/1 -> Out1/1
  Add/1 -> Add Delay - 2/1
  In1/1 -> Add/1
  J/1 -> Add/2

== system ensembleSNN_simulink/izhiekvichNeuron2/v' switch ==
  In1 : Inport
  In2 : Inport  Port=2
  In3 : Inport  Port=3
  Switch Delay - 3 : Delay  DelayLength=3
  Switch4 : Switch  Criteria=u2 > Threshold  Threshold=30
  J : Outport  VectorParamsAs1DForOutWhenUnconnected=on
  wires:
  In2/1 -> Switch4/2
  Switch4/1 -> Switch Delay - 3/1
  In1/1 -> Switch4/1
  Switch Delay - 3/1 -> J/1
  In3/1 -> Switch4/3

== system ensembleSNN_simulink/izhiekvichNeuron2/v^2 ==
  J : Inport
  In2 : Inport  Port=2
  Mult Delay - 2 : Delay  DelayLength=1
  Product1 : Product
  Out1 : Outport  VectorParamsAs1DForOutWhenUnconnected=on
  wires:
  Product1/1 -> Mult Delay - 2/1
  In2/1 -> Product1/2
  J/1 -> Product1/1
  Mult Delay - 2/1 -> Out1/1

== system ensembleSNN_simulink/izhiekvichNeuron3/0.04v2 +5v - u ==
  In1 : Inport
  In2 : Inport  Port=2
  Subtract : Sum  Inputs=+-
  Subtract Delay - 1 : Delay  DelayLength=1
  Out1 : Outport  VectorParamsAs1DForOutWhenUnconnected=on
  wires:
  In1/1 -> Subtract/1
  Subtract/1 -> Subtract Delay - 1/1
  Subtract Delay - 1/1 -> Out1/1
  In2/1 -> Subtract/2

== system ensembleSNN_simulink/izhiekvichNeuron3/0.04v2 +5v - u + j +140 ==
  In1 : Inport
  J : Inport  Port=2
  Add : Sum
  Add Delay - 2 : Delay
  Out1 : Outport  VectorParamsAs1DForOutWhenUnconnected=on
  wires:
  Add Delay - 2/1 -> Out1/1
  Add/1 -> Add Delay - 2/1
  In1/1 -> Add/1
  J/1 -> Add/2

== system ensembleSNN_simulink/izhiekvichNeuron3/0.04v^2 ==
  In1 : Inport
  In2 : Inport  Port=2
  Mult Delay - 1 : Delay  DelayLength=1
  Product1 : Product
  Out1 : Outport  VectorParamsAs1DForOutWhenUnconnected=on
  wires:
  Product1/1 -> Mult Delay - 1/1
  Mult Delay - 1/1 -> Out1/1
  In2/1 -> Product1/2
  In1/1 -> Product1/1

== system ensembleSNN_simulink/izhiekvichNeuron3/0.04v^2 +5v ==
  In1 : Inport
  In2 : Inport  Port=2
  Add : Sum
  Add Delay - 2 : Delay
  Out1 : Outport  VectorParamsAs1DForOutWhenUnconnected=on
  wires:
  Add Delay - 2/1 -> Out1/1
  Add/1 -> Add Delay - 2/1
  In1/1 -> Add/1
  In2/1 -> Add/2

== system ensembleSNN_simulink/izhiekvichNeuron3/5v ==
  J : Inport
  In2 : Inport  Port=2
  Mult Delay - 1 : Delay  DelayLength=1
  Product1 : Product
  Out1 : Outport  VectorParamsAs1DForOutWhenUnconnected=on
  wires:
  Product1/1 -> Mult Delay - 1/1
  Mult Delay - 1/1 -> Out1/1
  In2/1 -> Product1/2
  J/1 -> Product1/1

== system ensembleSNN_simulink/izhiekvichNeuron3/a(bv-u) ==
  In1 : Inport
  In2 : Inport  Port=2
  Mult Delay - 1 : Delay  DelayLength=1
  Product1 : Product
  Out1 : Outport  VectorParamsAs1DForOutWhenUnconnected=on
  wires:
  Product1/1 -> Mult Delay - 1/1
  Mult Delay - 1/1 -> Out1/1
  In2/1 -> Product1/2
  In1/1 -> Product1/1

== system ensembleSNN_simulink/izhiekvichNeuron3/bv ==
  In1 : Inport
  J : Inport  Port=2
  Mult Delay - 1 : Delay  DelayLength=1
  Product1 : Product
  Out1 : Outport  VectorParamsAs1DForOutWhenUnconnected=on
  wires:
  Product1/1 -> Mult Delay - 1/1
  Mult Delay - 1/1 -> Out1/1
  J/1 -> Product1/2
  In1/1 -> Product1/1

== system ensembleSNN_simulink/izhiekvichNeuron3/bv - u ==
  In1 : Inport
  In2 : Inport  Port=2
  Subtract : Sum  Inputs=+-
  Subtract Delay - 1 : Delay  DelayLength=1
  Out1 : Outport  VectorParamsAs1DForOutWhenUnconnected=on
  wires:
  In1/1 -> Subtract/1
  Subtract/1 -> Subtract Delay - 1/1
  Subtract Delay - 1/1 -> Out1/1
  In2/1 -> Subtract/2

== system ensembleSNN_simulink/izhiekvichNeuron3/j + 140 ==
  In1 : Inport
  J : Inport  Port=2
  Add : Sum
  Add Delay - 2 : Delay
  Out1 : Outport  VectorParamsAs1DForOutWhenUnconnected=on
  wires:
  Add Delay - 2/1 -> Out1/1
  Add/1 -> Add Delay - 2/1
  In1/1 -> Add/1
  J/1 -> Add/2

== system ensembleSNN_simulink/izhiekvichNeuron3/u + a(bv-u) ==
  In1 : Inport
  In2 : Inport  Port=2
  Add : Sum
  Add Delay - 2 : Delay
  Out1 : Outport  VectorParamsAs1DForOutWhenUnconnected=on
  wires:
  Add Delay - 2/1 -> Out1/1
  Add/1 -> Add Delay - 2/1
  In1/1 -> Add/1
  In2/1 -> Add/2

== system ensembleSNN_simulink/izhiekvichNeuron3/u' + d ==
  In1 : Inport
  In2 : Inport  Port=2
  Add : Sum
  Add Delay - 2 : Delay
  Out1 : Outport  VectorParamsAs1DForOutWhenUnconnected=on
  wires:
  Add Delay - 2/1 -> Out1/1
  Add/1 -> Add Delay - 2/1
  In1/1 -> Add/1
  In2/1 -> Add/2

== system ensembleSNN_simulink/izhiekvichNeuron3/u' switch ==
  In1 : Inport
  In2 : Inport  Port=2
  In3 : Inport  Port=3
  Switch Delay - 3 : Delay  DelayLength=3
  Switch4 : Switch  Criteria=u2 > Threshold  Threshold=30
  Out1 : Outport  VectorParamsAs1DForOutWhenUnconnected=on
  wires:
  In2/1 -> Switch4/2
  Switch4/1 -> Switch Delay - 3/1
  In1/1 -> Switch4/1
  Switch Delay - 3/1 -> Out1/1
  In3/1 -> Switch4/3

== system ensembleSNN_simulink/izhiekvichNeuron3/v + [0.04v2 +5v - u + j +140 ==
  In1 : Inport
  J : Inport  Port=2
  Add : Sum
  Add Delay - 2 : Delay
  Out1 : Outport  VectorParamsAs1DForOutWhenUnconnected=on
  wires:
  Add Delay - 2/1 -> Out1/1
  Add/1 -> Add Delay - 2/1
  In1/1 -> Add/1
  J/1 -> Add/2

== system ensembleSNN_simulink/izhiekvichNeuron3/v' switch ==
  In1 : Inport
  In2 : Inport  Port=2
  In3 : Inport  Port=3
  Switch Delay - 3 : Delay  DelayLength=3
  Switch4 : Switch  Criteria=u2 > Threshold  Threshold=30
  J : Outport  VectorParamsAs1DForOutWhenUnconnected=on
  wires:
  In2/1 -> Switch4/2
  Switch4/1 -> Switch Delay - 3/1
  In1/1 -> Switch4/1
  Switch Delay - 3/1 -> J/1
  In3/1 -> Switch4/3

== system ensembleSNN_simulink/izhiekvichNeuron3/v^2 ==
  J : Inport
  In2 : Inport  Port=2
  Mult Delay - 2 : Delay  DelayLength=1
  Product1 : Product
  Out1 : Outport  VectorParamsAs1DForOutWhenUnconnected=on
  wires:
  Product1/1 -> Mult Delay - 2/1
  In2/1 -> Product1/2
  J/1 -> Product1/1
  Mult Delay - 2/1 -> Out1/1

== system ensembleSNN_simulink/izhiekvichNeuron4/0.04v2 +5v - u ==
  In1 : Inport
  In2 : Inport  Port=2
  Subtract : Sum  Inputs=+-
  Subtract Delay - 1 : Delay  DelayLength=1
  Out1 : Outport  VectorParamsAs1DForOutWhenUnconnected=on
  wires:
  In1/1 -> Subtract/1
  Subtract/1 -> Subtract Delay - 1/1
  Subtract Delay - 1/1 -> Out1/1
  In2/1 -> Subtract/2

== system ensembleSNN_simulink/izhiekvichNeuron4/0.04v2 +5v - u + j +140 ==
  In1 : Inport
  J : Inport  Port=2
  Add : Sum
  Add Delay - 2 : Delay
  Out1 : Outport  VectorParamsAs1DForOutWhenUnconnected=on
  wires:
  Add Delay - 2/1 -> Out1/1
  Add/1 -> Add Delay - 2/1
  In1/1 -> Add/1
  J/1 -> Add/2

== system ensembleSNN_simulink/izhiekvichNeuron4/0.04v^2 ==
  In1 : Inport
  In2 : Inport  Port=2
  Mult Delay - 1 : Delay  DelayLength=1
  Product1 : Product
  Out1 : Outport  VectorParamsAs1DForOutWhenUnconnected=on
  wires:
  Product1/1 -> Mult Delay - 1/1
  Mult Delay - 1/1 -> Out1/1
  In2/1 -> Product1/2
  In1/1 -> Product1/1

== system ensembleSNN_simulink/izhiekvichNeuron4/0.04v^2 +5v ==
  In1 : Inport
  In2 : Inport  Port=2
  Add : Sum
  Add Delay - 2 : Delay
  Out1 : Outport  VectorParamsAs1DForOutWhenUnconnected=on
  wires:
  Add Delay - 2/1 -> Out1/1
  Add/1 -> Add Delay - 2/1
  In1/1 -> Add/1
  In2/1 -> Add/2

== system ensembleSNN_simulink/izhiekvichNeuron4/5v ==
  J : Inport
  In2 : Inport  Port=2
  Mult Delay - 1 : Delay  DelayLength=1
  Product1 : Product
  Out1 : Outport  VectorParamsAs1DForOutWhenUnconnected=on
  wires:
  Product1/1 -> Mult Delay - 1/1
  Mult Delay - 1/1 -> Out1/1
  In2/1 -> Product1/2
  J/1 -> Product1/1

== system ensembleSNN_simulink/izhiekvichNeuron4/a(bv-u) ==
  In1 : Inport
  In2 : Inport  Port=2
  Mult Delay - 1 : Delay  DelayLength=1
  Product1 : Product
  Out1 : Outport  VectorParamsAs1DForOutWhenUnconnected=on
  wires:
  Product1/1 -> Mult Delay - 1/1
  Mult Delay - 1/1 -> Out1/1
  In2/1 -> Product1/2
  In1/1 -> Product1/1

== system ensembleSNN_simulink/izhiekvichNeuron4/bv ==
  In1 : Inport
  J : Inport  Port=2
  Mult Delay - 1 : Delay  DelayLength=1
  Product1 : Product
  Out1 : Outport  VectorParamsAs1DForOutWhenUnconnected=on
  wires:
  Product1/1 -> Mult Delay - 1/1
  Mult Delay - 1/1 -> Out1/1
  J/1 -> Product1/2
  In1/1 -> Product1/1

== system ensembleSNN_simulink/izhiekvichNeuron4/bv - u ==
  In1 : Inport
  In2 : Inport  Port=2
  Subtract : Sum  Inputs=+-
  Subtract Delay - 1 : Delay  DelayLength=1
  Out1 : Outport  VectorParamsAs1DForOutWhenUnconnected=on
  wires:
  In1/1 -> Subtract/1
  Subtract/1 -> Subtract Delay - 1/1
  Subtract Delay - 1/1 -> Out1/1
  In2/1 -> Subtract/2

== system ensembleSNN_simulink/izhiekvichNeuron4/j + 140 ==
  In1 : Inport
  J : Inport  Port=2
  Add : Sum
  Add Delay - 2 : Delay
  Out1 : Outport  VectorParamsAs1DForOutWhenUnconnected=on
  wires:
  Add Delay - 2/1 -> Out1/1
  Add/1 -> Add Delay - 2/1
  In1/1 -> Add/1
  J/1 -> Add/2

== system ensembleSNN_simulink/izhiekvichNeuron4/u + a(bv-u) ==
  In1 : Inport
  In2 : Inport  Port=2
  Add : Sum
  Add Delay - 2 : Delay
  Out1 : Outport  VectorParamsAs1DForOutWhenUnconnected=on
  wires:
  Add Delay - 2/1 -> Out1/1
  Add/1 -> Add Delay - 2/1
  In1/1 -> Add/1
  In2/1 -> Add/2

== system ensembleSNN_simulink/izhiekvichNeuron4/u' + d ==
  In1 : Inport
  In2 : Inport  Port=2
  Add : Sum
  Add Delay - 2 : Delay
  Out1 : Outport  VectorParamsAs1DForOutWhenUnconnected=on
  wires:
  Add Delay - 2/1 -> Out1/1
  Add/1 -> Add Delay - 2/1
  In1/1 -> Add/1
  In2/1 -> Add/2

== system ensembleSNN_simulink/izhiekvichNeuron4/u' switch ==
  In1 : Inport
  In2 : Inport  Port=2
  In3 : Inport  Port=3
  Switch Delay - 3 : Delay  DelayLength=3
  Switch4 : Switch  Criteria=u2 > Threshold  Threshold=30
  Out1 : Outport  VectorParamsAs1DForOutWhenUnconnected=on
  wires:
  In2/1 -> Switch4/2
  Switch4/1 -> Switch Delay - 3/1
  In1/1 -> Switch4/1
  Switch Delay - 3/1 -> Out1/1
  In3/1 -> Switch4/3

== system ensembleSNN_simulink/izhiekvichNeuron4/v + [0.04v2 +5v - u + j +140 ==
  In1 : Inport
  J : Inport  Port=2
  Add : Sum
  Add Delay - 2 : Delay
  Out1 : Outport  VectorParamsAs1DForOutWhenUnconnected=on
  wires:
  Add Delay - 2/1 -> Out1/1
  Add/1 -> Add Delay - 2/1
  In1/1 -> Add/1
  J/1 -> Add/2

== system ensembleSNN_simulink/izhiekvichNeuron4/v' switch ==
  In1 : Inport
  In2 : Inport  Port=2
  In3 : Inport  Port=3
  Switch Delay - 3 : Delay  DelayLength=3
  Switch4 : Switch  Criteria=u2 > Threshold  Threshold=30
  J : Outport  VectorParamsAs1DForOutWhenUnconnected=on
  wires:
  In2/1 -> Switch4/2
  Switch4/1 -> Switch Delay - 3/1
  In1/1 -> Switch4/1
  Switch Delay - 3/1 -> J/1
  In3/1 -> Switch4/3

== system ensembleSNN_simulink/izhiekvichNeuron4/v^2 ==
  J : Inport
  In2 : Inport  Port=2
  Mult Delay - 2 : Delay  DelayLength=1
  Product1 : Product
  Out1 : Outport  VectorParamsAs1DForOutWhenUnconnected=on
  wires:
  Product1/1 -> Mult Delay - 2/1
  In2/1 -> Product1/2
  J/1 -> Product1/1
  Mult Delay - 2/1 -> Out1/1

== system ensembleSNN_simulink/izhiekvichNeuron5/0.04v2 +5v - u ==
  In1 : Inport
  In2 : Inport  Port=2
  Subtract : Sum  Inputs=+-
  Subtract Delay - 1 : Delay  DelayLength=1
  Out1 : Outport  VectorParamsAs1DForOutWhenUnconnected=on
  wires:
  In1/1 -> Subtract/1
  Subtract/1 -> Subtract Delay - 1/1
  Subtract Delay - 1/1 -> Out1/1
  In2/1 -> Subtract/2

== system ensembleSNN_simulink/izhiekvichNeuron5/0.04v2 +5v - u + j +140 ==
  In1 : Inport
  J : Inport  Port=2
  Add : Sum
  Add Delay - 2 : Delay
  Out1 : Outport  VectorParamsAs1DForOutWhenUnconnected=on
  wires:
  Add Delay - 2/1 -> Out1/1
  Add/1 -> Add Delay - 2/1
  In1/1 -> Add/1
  J/1 -> Add/2

== system ensembleSNN_simulink/izhiekvichNeuron5/0.04v^2 ==
  In1 : Inport
  In2 : Inport  Port=2
  Mult Delay - 1 : Delay  DelayLength=1
  Product1 : Product
  Out1 : Outport  VectorParamsAs1DForOutWhenUnconnected=on
  wires:
  Product1/1 -> Mult Delay - 1/1
  Mult Delay - 1/1 -> Out1/1
  In2/1 -> Product1/2
  In1/1 -> Product1/1

== system ensembleSNN_simulink/izhiekvichNeuron5/0.04v^2 +5v ==
  In1 : Inport
  In2 : Inport  Port=2
  Add : Sum
  Add Delay - 2 : Delay
  Out1 : Outport  VectorParamsAs1DForOutWhenUnconnected=on
  wires:
  Add Delay - 2/1 -> Out1/1
  Add/1 -> Add Delay - 2/1
  In1/1 -> Add/1
  In2/1 -> Add/2

== system ensembleSNN_simulink/izhiekvichNeuron5/5v ==
  J : Inport
  In2 : Inport  Port=2
  Mult Delay - 1 : Delay  DelayLength=1
  Product1 : Product
  Out1 : Outport  VectorParamsAs1DForOutWhenUnconnected=on
  wires:
  Product1/1 -> Mult Delay - 1/1
  Mult Delay - 1/1 -> Out1/1
  In2/1 -> Product1/2
  J/1 -> Product1/1

== system ensembleSNN_simulink/izhiekvichNeuron5/a(bv-u) ==
  In1 : Inport
  In2 : Inport  Port=2
  Mult Delay - 1 : Delay  DelayLength=1
  Product1 : Product
  Out1 : Outport  VectorParamsAs1DForOutWhenUnconnected=on
  wires:
  Product1/1 -> Mult Delay - 1/1
  Mult Delay - 1/1 -> Out1/1
  In2/1 -> Product1/2
  In1/1 -> Product1/1

== system ensembleSNN_simulink/izhiekvichNeuron5/bv ==
  In1 : Inport
  J : Inport  Port=2
  Mult Delay - 1 : Delay  DelayLength=1
  Product1 : Product
  Out1 : Outport  VectorParamsAs1DForOutWhenUnconnected=on
  wires:
  Product1/1 -> Mult Delay - 1/1
  Mult Delay - 1/1 -> Out1/1
  J/1 -> Product1/2
  In1/1 -> Product1/1

== system ensembleSNN_simulink/izhiekvichNeuron5/bv - u ==
  In1 : Inport
  In2 : Inport  Port=2
  Subtract : Sum  Inputs=+-
  Subtract Delay - 1 : Delay  DelayLength=1
  Out1 : Outport  VectorParamsAs1DForOutWhenUnconnected=on
  wires:
  In1/1 -> Subtract/1
  Subtract/1 -> Subtract Delay - 1/1
  Subtract Delay - 1/1 -> Out1/1
  In2/1 -> Subtract/2

== system ensembleSNN_simulink/izhiekvichNeuron5/j + 140 ==
  In1 : Inport
  J : Inport  Port=2
  Add : Sum
  Add Delay - 2 : Delay
  Out1 : Outport  VectorParamsAs1DForOutWhenUnconnected=on
  wires:
  Add Delay - 2/1 -> Out1/1
  Add/1 -> Add Delay - 2/1
  In1/1 -> Add/1
  J/1 -> Add/2

== system ensembleSNN_simulink/izhiekvichNeuron5/u + a(bv-u) ==
  In1 : Inport
  In2 : Inport  Port=2
  Add : Sum
  Add Delay - 2 : Delay
  Out1 : Outport  VectorParamsAs1DForOutWhenUnconnected=on
  wires:
  Add Delay - 2/1 -> Out1/1
  Add/1 -> Add Delay - 2/1
  In1/1 -> Add/1
  In2/1 -> Add/2

== system ensembleSNN_simulink/izhiekvichNeuron5/u' + d ==
  In1 : Inport
  In2 : Inport  Port=2
  Add : Sum
  Add Delay - 2 : Delay
  Out1 : Outport  VectorParamsAs1DForOutWhenUnconnected=on
  wires:
  Add Delay - 2/1 -> Out1/1
  Add/1 -> Add Delay - 2/1
  In1/1 -> Add/1
  In2/1 -> Add/2

== system ensembleSNN_simulink/izhiekvichNeuron5/u' switch ==
  In1 : Inport
  In2 : Inport  Port=2
  In3 : Inport  Port=3
  Switch Delay - 3 : Delay  DelayLength=3
  Switch4 : Switch  Criteria=u2 > Threshold  Threshold=30
  Out1 : Outport  VectorParamsAs1DForOutWhenUnconnected=on
  wires:
  In2/1 -> Switch4/2
  Switch4/1 -> Switch Delay - 3/1
  In1/1 -> Switch4/1
  Switch Delay - 3/1 -> Out1/1
  In3/1 -> Switch4/3

== system ensembleSNN_simulink/izhiekvichNeuron5/v + [0.04v2 +5v - u + j +140 ==
  In1 : Inport
  J : Inport  Port=2
  Add : Sum
  Add Delay - 2 : Delay
  Out1 : Outport  VectorParamsAs1DForOutWhenUnconnected=on
  wires:
  Add Delay - 2/1 -> Out1/1
  Add/1 -> Add Delay - 2/1
  In1/1 -> Add/1
  J/1 -> Add/2

== system ensembleSNN_simulink/izhiekvichNeuron5/v' switch ==
  In1 : Inport
  In2 : Inport  Port=2
  In3 : Inport  Port=3
  Switch Delay - 3 : Delay  DelayLength=3
  Switch4 : Switch  Criteria=u2 > Threshold  Threshold=30
  J : Outport  VectorParamsAs1DForOutWhenUnconnected=on
  wires:
  In2/1 -> Switch4/2
  Switch4/1 -> Switch Delay - 3/1
  In1/1 -> Switch4/1
  Switch Delay - 3/1 -> J/1
  In3/1 -> Switch4/3

== system ensembleSNN_simulink/izhiekvichNeuron5/v^2 ==
  J : Inport
  In2 : Inport  Port=2
  Mult Delay - 2 : Delay  DelayLength=1
  Product1 : Product
  Out1 : Outport  VectorParamsAs1DForOutWhenUnconnected=on
  wires:
  Product1/1 -> Mult Delay - 2/1
  In2/1 -> Product1/2
  J/1 -> Product1/1
  Mult Delay - 2/1 -> Out1/1

== system ensembleSNN_simulink/izhiekvichNeuron6/0.04v2 +5v - u ==
  In1 : Inport
  In2 : Inport  Port=2
  Subtract : Sum  Inputs=+-
  Subtract Delay - 1 : Delay  DelayLength=1
  Out1 : Outport  VectorParamsAs1DForOutWhenUnconnected=on
  wires:
  In1/1 -> Subtract/1
  Subtract/1 -> Subtract Delay - 1/1
  Subtract Delay - 1/1 -> Out1/1
  In2/1 -> Subtract/2

== system ensembleSNN_simulink/izhiekvichNeuron6/0.04v2 +5v - u + j +140 ==
  In1 : Inport
  J : Inport  Port=2
  Add : Sum
  Add Delay - 2 : Delay
  Out1 : Outport  VectorParamsAs1DForOutWhenUnconnected=on
  wires:
  Add Delay - 2/1 -> Out1/1
  Add/1 -> Add Delay - 2/1
  In1/1 -> Add/1
  J/1 -> Add/2

== system ensembleSNN_simulink/izhiekvichNeuron6/0.04v^2 ==
  In1 : Inport
  In2 : Inport  Port=2
  Mult Delay - 1 : Delay  DelayLength=1
  Product1 : Product
  Out1 : Outport  VectorParamsAs1DForOutWhenUnconnected=on
  wires:
  Product1/1 -> Mult Delay - 1/1
  Mult Delay - 1/1 -> Out1/1
  In2/1 -> Product1/2
  In1/1 -> Product1/1

== system ensembleSNN_simulink/izhiekvichNeuron6/0.04v^2 +5v ==
  In1 : Inport
  In2 : Inport  Port=2
  Add : Sum
  Add Delay - 2 : Delay
  Out1 : Outport  VectorParamsAs1DForOutWhenUnconnected=on
  wires:
  Add Delay - 2/1 -> Out1/1
  Add/1 -> Add Delay - 2/1
  In1/1 -> Add/1
  In2/1 -> Add/2

== system ensembleSNN_simulink/izhiekvichNeuron6/5v ==
  J : Inport
  In2 : Inport  Port=2
  Mult Delay - 1 : Delay  DelayLength=1
  Product1 : Product
  Out1 : Outport  VectorParamsAs1DForOutWhenUnconnected=on
  wires:
  Product1/1 -> Mult Delay - 1/1
  Mult Delay - 1/1 -> Out1/1
  In2/1 -> Product1/2
  J/1 -> Product1/1

== system ensembleSNN_simulink/izhiekvichNeuron6/a(bv-u) ==
  In1 : Inport
  In2 : Inport  Port=2
  Mult Delay - 1 : Delay  DelayLength=1
  Product1 : Product
  Out1 : Outport  VectorParamsAs1DForOutWhenUnconnected=on
  wires:
  Product1/1 -> Mult Delay - 1/1
  Mult Delay - 1/1 -> Out1/1
  In2/1 -> Product1/2
  In1/1 -> Product1/1

== system ensembleSNN_simulink/izhiekvichNeuron6/bv ==
  In1 : Inport
  J : Inport  Port=2
  Mult Delay - 1 : Delay  DelayLength=1
  Product1 : Product
  Out1 : Outport  VectorParamsAs1DForOutWhenUnconnected=on
  wires:
  Product1/1 -> Mult Delay - 1/1
  Mult Delay - 1/1 -> Out1/1
  J/1 -> Product1/2
  In1/1 -> Product1/1

== system ensembleSNN_simulink/izhiekvichNeuron6/bv - u ==
  In1 : Inport
  In2 : Inport  Port=2
  Subtract : Sum  Inputs=+-
  Subtract Delay - 1 : Delay  DelayLength=1
  Out1 : Outport  VectorParamsAs1DForOutWhenUnconnected=on
  wires:
  In1/1 -> Subtract/1
  Subtract/1 -> Subtract Delay - 1/1
  Subtract Delay - 1/1 -> Out1/1
  In2/1 -> Subtract/2

== system ensembleSNN_simulink/izhiekvichNeuron6/j + 140 ==
  In1 : Inport
  J : Inport  Port=2
  Add : Sum
  Add Delay - 2 : Delay
  Out1 : Outport  VectorParamsAs1DForOutWhenUnconnected=on
  wires:
  Add Delay - 2/1 -> Out1/1
  Add/1 -> Add Delay - 2/1
  In1/1 -> Add/1
  J/1 -> Add/2

== system ensembleSNN_simulink/izhiekvichNeuron6/u + a(bv-u) ==
  In1 : Inport
  In2 : Inport  Port=2
  Add : Sum
  Add Delay - 2 : Delay
  Out1 : Outport  VectorParamsAs1DForOutWhenUnconnected=on
  wires:
  Add Delay - 2/1 -> Out1/1
  Add/1 -> Add Delay - 2/1
  In1/1 -> Add/1
  In2/1 -> Add/2

== system ensembleSNN_simulink/izhiekvichNeuron6/u' + d ==
  In1 : Inport
  In2 : Inport  Port=2
  Add : Sum
  Add Delay - 2 : Delay
  Out1 : Outport  VectorParamsAs1DForOutWhenUnconnected=on
  wires:
  Add Delay - 2/1 -> Out1/1
  Add/1 -> Add Delay - 2/1
  In1/1 -> Add/1
  In2/1 -> Add/2
